simulink model "lab32"  (R2021a)
settings: Solver=VariableStepAuto  StartTime=0.0  StopTime=1  RelTol=1e-3
settings Model: Creator=asr77  LastModifiedBy=asr77

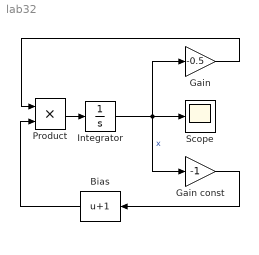
== system lab32 ==
  "Bias " : Bias  Bias=1
  "Gain " : Gain  Gain=-0.5
  Gain const : Gain  Gain=-1
  "Integrator " : Integrator  InitialCondition=1.01:0.2:2.01
  "Product " : Product
  "Scope " : Scope
  wires:
  "Integrator "/1 -> "Scope "/1, "Gain "/1, Gain const/1  "x"
  Gain const/1 -> "Bias "/1
  "Product "/1 -> "Integrator "/1
  "Bias "/1 -> "Product "/2
  "Gain "/1 -> "Product "/1
